simulink model "LTI_1st_older"  (R2020a)
settings: Solver=VariableStepAuto  StartTime=0.0  StopTime=10.0  RelTol=1e-3
settings Model: Creator=BUAA_CZF  LastModifiedBy=BUAA_CZF

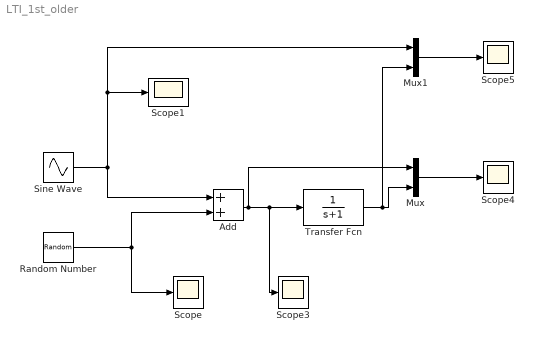
== system LTI_1st_older ==
  Add : Sum
  Mux : Mux  Inputs=2
  Mux1 : Mux  Inputs=2
  "Random Number " : RandomNumber  Variance=0.1  SampleTime=0.01
  Scope{,1,3..5} (5 alike) : Scope
  "Sine Wave " : Sin  SampleTime=0
  "Transfer Fcn " : TransferFcn  Denominator=[1 1]
  wires:
  "Random Number "/1 -> Scope/1, Add/2
  Add/1 -> Mux/1, Scope3/1, "Transfer Fcn "/1
  Mux/1 -> Scope4/1
  Mux1/1 -> Scope5/1
  "Sine Wave "/1 -> Mux1/1, Scope1/1, Add/1
  "Transfer Fcn "/1 -> Mux1/2, Mux/2
